simulink subsystem "ergocub_head"  (R2026a)
settings: Solver=VariableStepAuto
undefined symbols (not defined in the file): ergoCubHead_mass_scale, ergoCubHeadData, headData, X, Y, Z
libraries: sm_lib x10
settings Model: DataDictionary=ergocub_head_data.sldd  EnableAccessToBaseWorkspace=off  Creator=upattacini  LastModifiedBy=upattacini

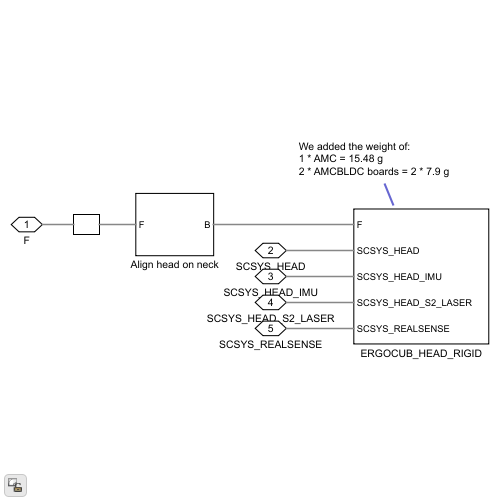
[thumbnail: Simulink's stored preview of the top-level diagram]
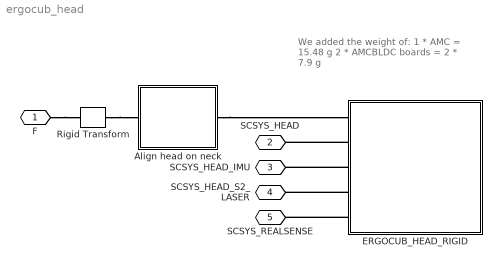
== system ergocub_head ==
  note: We added the weight of:
      | 1 * AMC = 15.48 g
      | 2 * AMCBLDC boards = 2 * 7.9 g
  Align head on neck : Subsystem
  ERGOCUB_HEAD_RIGID : Subsystem
  Rigid Transform : sm_lib/Frames and Transforms/Rigid Transform  RotationMethod=None  FollAlignAxisA=+X  BaseAlignAxisA=+Y  FollAlignAxisB=+Y  BaseAlignAxisB=+Z  RotationStandardAxis=+Z  RotationAngle=0  RotationAngleUnits=deg  RotationArbitraryAxis=[0 0 1]  RotationSequenceAxes=FollowerAxes  RotationSequence=XYX  RotationSequenceAngles=[0 0 0]  RotationSequenceAnglesUnits=deg  RotationMatrix=[1 0 0;0 1 0;0 0 1]  Quaternion=[1 0 0 0]  TranslationMethod=StandardAxis  TranslationCartesianOffset=[0 0 0]  TranslationCartesianOffsetUnits=m  TranslationStandardAxis=+Y  TranslationStandardOffset=ergoCubHead_z_offset  TranslationStandardOffsetUnits=mm  TranslationROffset=0  TranslationROffsetUnits=m  TranslationThetaOffset=0  TranslationThetaOffsetUnits=deg  TranslationZOffset=0  TranslationZOffsetUnits=m
  F : PMIOPort  Side=Left
  SCSYS_HEAD : PMIOPort  Port=2  Side=Left
  SCSYS_HEAD_IMU : PMIOPort  Port=3  Side=Left
  SCSYS_HEAD_S2_LASER : PMIOPort  Port=4  Side=Left
  SCSYS_REALSENSE : PMIOPort  Port=5  Side=Left
  connections:
  Align head on neck/LConn1 -- ERGOCUB_HEAD_RIGID/LConn1
  ERGOCUB_HEAD_RIGID/LConn5 -- SCSYS_REALSENSE/RConn1
  ERGOCUB_HEAD_RIGID/LConn4 -- SCSYS_HEAD_S2_LASER/RConn1
  Rigid Transform/RConn1 -- Align head on neck/RConn1
  ERGOCUB_HEAD_RIGID/LConn3 -- SCSYS_HEAD_IMU/RConn1
  ERGOCUB_HEAD_RIGID/LConn2 -- SCSYS_HEAD/RConn1
  F/RConn1 -- Rigid Transform/LConn1

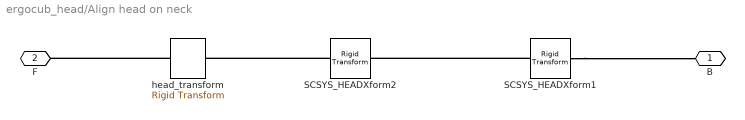
== system ergocub_head/Align head on neck ==
  SCSYS_HEADXform1 : sm_lib/Frames and Transforms/Rigid Transform  RotationMethod=ArbitraryAxis  FollAlignAxisA=+X  BaseAlignAxisA=+Y  FollAlignAxisB=+Y  BaseAlignAxisB=+Z  RotationStandardAxis=+Z  RotationAngle=ergoCubHeadData.RigidTransform(2).angle  RotationAngleUnits=rad  RotationArbitraryAxis=ergoCubHeadData.RigidTransform(2).axis  RotationSequenceAxes=FollowerAxes  RotationSequence=XYX  RotationSequenceAngles=[0 0 0]  RotationSequenceAnglesUnits=deg  RotationMatrix=[1 0 0; 0 1 0; 0 0 1]  Quaternion=[1 0 0 0]  TranslationMethod=Cartesian  TranslationCartesianOffset=ergoCubHeadData.RigidTransform(2).translation  TranslationCartesianOffsetUnits=mm  TranslationStandardAxis=+Z  TranslationStandardOffset=0  TranslationStandardOffsetUnits=mm  TranslationROffset=0  TranslationROffsetUnits=m  TranslationThetaOffset=0  TranslationThetaOffsetUnits=deg  TranslationZOffset=0  TranslationZOffsetUnits=m
  SCSYS_HEADXform2 : sm_lib/Frames and Transforms/Rigid Transform  RotationMethod=RotationSequence  FollAlignAxisA=+X  BaseAlignAxisA=+Y  FollAlignAxisB=+Y  BaseAlignAxisB=+Z  RotationStandardAxis=+Z  RotationAngle=headData.RigidTransform(4).angle  RotationAngleUnits=rad  RotationArbitraryAxis=headData.RigidTransform(4).axis  RotationSequenceAxes=FollowerAxes  RotationSequence=XYZ  RotationSequenceAngles=[-90 90 0]  RotationSequenceAnglesUnits=deg  RotationMatrix=[1 0 0; 0 1 0; 0 0 1]  Quaternion=[1 0 0 0]  TranslationMethod=None  TranslationCartesianOffset=[0 0 -78.65]  TranslationCartesianOffsetUnits=mm  TranslationStandardAxis=+Z  TranslationStandardOffset=0  TranslationStandardOffsetUnits=mm  TranslationROffset=0  TranslationROffsetUnits=m  TranslationThetaOffset=0  TranslationThetaOffsetUnits=deg  TranslationZOffset=0  TranslationZOffsetUnits=m
  head_transform : sm_lib/Frames and Transforms/Rigid Transform  RotationMethod=RotationSequence  FollAlignAxisA=+X  BaseAlignAxisA=+Y  FollAlignAxisB=+Y  BaseAlignAxisB=+Z  RotationStandardAxis=+Z  RotationAngle=0.0  RotationAngleUnits=deg  RotationArbitraryAxis=[0 0 1]  RotationSequenceAxes=FollowerAxes  RotationSequence=XYX  RotationSequenceAngles=[180 90 0]  RotationSequenceAnglesUnits=deg  RotationMatrix=[1 0 0; 0 1 0; 0 0 1]  Quaternion=[1 0 0 0]  TranslationMethod=Cartesian  TranslationCartesianOffset=[0 3 0]  TranslationCartesianOffsetUnits=mm  TranslationStandardAxis=+Z  TranslationStandardOffset=0  TranslationStandardOffsetUnits=mm  TranslationROffset=0  TranslationROffsetUnits=m  TranslationThetaOffset=0  TranslationThetaOffsetUnits=deg  TranslationZOffset=0  TranslationZOffsetUnits=m
  B : PMIOPort  Side=Left
  F : PMIOPort  Port=2  Side=Right
  connections:
  SCSYS_HEADXform2/RConn1 -- head_transform/RConn1
  SCSYS_HEADXform1/LConn1 -- B/RConn1
  head_transform/LConn1 -- F/RConn1
  SCSYS_HEADXform1/RConn1 -- SCSYS_HEADXform2/LConn1

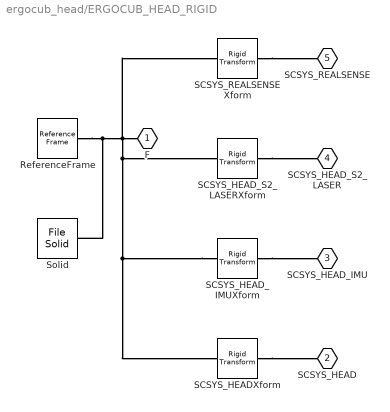
== system ergocub_head/ERGOCUB_HEAD_RIGID ==
  ReferenceFrame : sm_lib/Frames and Transforms/Reference Frame
  SCSYS_HEADXform : sm_lib/Frames and Transforms/Rigid Transform  RotationMethod=ArbitraryAxis  FollAlignAxisA=+X  BaseAlignAxisA=+Y  FollAlignAxisB=+Y  BaseAlignAxisB=+Z  RotationStandardAxis=+Z  RotationAngle=ergoCubHeadData.RigidTransform(2).angle  RotationAngleUnits=rad  RotationArbitraryAxis=ergoCubHeadData.RigidTransform(2).axis  RotationSequenceAxes=FollowerAxes  RotationSequence=XYX  RotationSequenceAngles=[0 0 0]  RotationSequenceAnglesUnits=deg  RotationMatrix=[1 0 0; 0 1 0; 0 0 1]  Quaternion=[1 0 0 0]  TranslationMethod=Cartesian  TranslationCartesianOffset=ergoCubHeadData.RigidTransform(2).translation  TranslationCartesianOffsetUnits=mm  TranslationStandardAxis=+Z  TranslationStandardOffset=0  TranslationStandardOffsetUnits=mm  TranslationROffset=0  TranslationROffsetUnits=m  TranslationThetaOffset=0  TranslationThetaOffsetUnits=deg  TranslationZOffset=0  TranslationZOffsetUnits=m
  SCSYS_HEAD_IMUXform : sm_lib/Frames and Transforms/Rigid Transform  RotationMethod=ArbitraryAxis  FollAlignAxisA=+X  BaseAlignAxisA=+Y  FollAlignAxisB=+Y  BaseAlignAxisB=+Z  RotationStandardAxis=+Z  RotationAngle=ergoCubHeadData.RigidTransform(4).angle  RotationAngleUnits=rad  RotationArbitraryAxis=ergoCubHeadData.RigidTransform(4).axis  RotationSequenceAxes=FollowerAxes  RotationSequence=XYX  RotationSequenceAngles=[0 0 0]  RotationSequenceAnglesUnits=deg  RotationMatrix=[1 0 0; 0 1 0; 0 0 1]  Quaternion=[1 0 0 0]  TranslationMethod=Cartesian  TranslationCartesianOffset=ergoCubHeadData.RigidTransform(4).translation  TranslationCartesianOffsetUnits=mm  TranslationStandardAxis=+Z  TranslationStandardOffset=0  TranslationStandardOffsetUnits=mm  TranslationROffset=0  TranslationROffsetUnits=m  TranslationThetaOffset=0  TranslationThetaOffsetUnits=deg  TranslationZOffset=0  TranslationZOffsetUnits=m
  SCSYS_HEAD_S2_LASERXform : sm_lib/Frames and Transforms/Rigid Transform  RotationMethod=ArbitraryAxis  FollAlignAxisA=+X  BaseAlignAxisA=+Y  FollAlignAxisB=+Y  BaseAlignAxisB=+Z  RotationStandardAxis=+Z  RotationAngle=ergoCubHeadData.RigidTransform(3).angle  RotationAngleUnits=rad  RotationArbitraryAxis=ergoCubHeadData.RigidTransform(3).axis  RotationSequenceAxes=FollowerAxes  RotationSequence=XYX  RotationSequenceAngles=[0 0 0]  RotationSequenceAnglesUnits=deg  RotationMatrix=[1 0 0; 0 1 0; 0 0 1]  Quaternion=[1 0 0 0]  TranslationMethod=Cartesian  TranslationCartesianOffset=ergoCubHeadData.RigidTransform(3).translation  TranslationCartesianOffsetUnits=mm  TranslationStandardAxis=+Z  TranslationStandardOffset=0  TranslationStandardOffsetUnits=mm  TranslationROffset=0  TranslationROffsetUnits=m  TranslationThetaOffset=0  TranslationThetaOffsetUnits=deg  TranslationZOffset=0  TranslationZOffsetUnits=m
  SCSYS_REALSENSEXform : sm_lib/Frames and Transforms/Rigid Transform  RotationMethod=ArbitraryAxis  FollAlignAxisA=+X  BaseAlignAxisA=+Y  FollAlignAxisB=+Y  BaseAlignAxisB=+Z  RotationStandardAxis=+Z  RotationAngle=ergoCubHeadData.RigidTransform(1).angle  RotationAngleUnits=rad  RotationArbitraryAxis=ergoCubHeadData.RigidTransform(1).axis  RotationSequenceAxes=FollowerAxes  RotationSequence=XYX  RotationSequenceAngles=[0 0 0]  RotationSequenceAnglesUnits=deg  RotationMatrix=[1 0 0; 0 1 0; 0 0 1]  Quaternion=[1 0 0 0]  TranslationMethod=Cartesian  TranslationCartesianOffset=ergoCubHeadData.RigidTransform(1).translation  TranslationCartesianOffsetUnits=mm  TranslationStandardAxis=+Z  TranslationStandardOffset=0  TranslationStandardOffsetUnits=mm  TranslationROffset=0  TranslationROffsetUnits=m  TranslationThetaOffset=0  TranslationThetaOffsetUnits=deg  TranslationZOffset=0  TranslationZOffsetUnits=m
  Solid : sm_lib/Body Elements/File Solid  ExtGeomFileName=ergocub_head_prt.step  UnitType=FromFile  ExtGeomFileUnits=m  StepReaderType=HEX  ExportConvexHullGeometry=off  InertiaType=Custom  BasedOnType=DensityFromFile  Density=1000  DensityUnits=kg/m^3  Mass=ergoCubHead_mass_scale*ergoCubHeadData.Solid(1).mass  MassUnits=kg  CenterOfMass=ergoCubHeadData.Solid(1).CoM  CenterOfMassUnits=mm  MomentsOfInertia=ergoCubHead_mass_scale*ergoCubHeadData.Solid(1).MoI  MomentsOfInertiaUnits=kg*mm^2  ProductsOfInertia=ergoCubHead_mass_scale*ergoCubHeadData.Solid(1).PoI  ProductsOfInertiaUnits=kg*mm^2  GraphicType=FromGeometry  MarkerShape=Sphere  MarkerSize=10  GraphicVisPropType=SimpleVisualProperties  GraphicDiffuseColor=ergoCubHeadData.Solid(1).color  GraphicOpacity=ergoCubHeadData.Solid(1).opacity  GraphicSpecularColor=[0.5 0.5 0.5 1.0]  GraphicAmbientColor=[0.15 0.15 0.15 1.0]  GraphicEmissiveColor=[0.0 0.0 0.0 1.0]  GraphicShininess=75  DoExposeReferenceFrame=on  SerializedFrames=<Frames/>
  F : PMIOPort  Side=Left
  SCSYS_HEAD : PMIOPort  Port=2  Side=Left
  SCSYS_HEAD_IMU : PMIOPort  Port=3  Side=Left
  SCSYS_HEAD_S2_LASER : PMIOPort  Port=4  Side=Left
  SCSYS_REALSENSE : PMIOPort  Port=5  Side=Left
  connections:
  SCSYS_HEAD_IMUXform/RConn1 -- SCSYS_HEAD_IMU/RConn1
  SCSYS_HEAD_S2_LASERXform/RConn1 -- SCSYS_HEAD_S2_LASER/RConn1
  SCSYS_HEADXform/RConn1 -- SCSYS_HEAD/RConn1
  SCSYS_REALSENSEXform/RConn1 -- SCSYS_REALSENSE/RConn1
  SCSYS_HEAD_IMUXform/LConn1 -- SCSYS_HEAD_S2_LASERXform/LConn1 -- F/RConn1 -- SCSYS_REALSENSEXform/LConn1 -- Solid/RConn1 -- ReferenceFrame/RConn1 -- SCSYS_HEADXform/LConn1
